simulink model "Aktuator"  (R2019b)
settings: Solver=FixedStepAuto  StartTime=0.0  StopTime=2  FixedStep=0.00001  RelTol=1e-3
values from neighbouring files (symbols this model uses):
  Drehzahlkonstante = 1070    [Init_Aktuator.m]    (also in Init_Aktuator_Klapp.m = 569; Init_Aktuator_Steuer.m)
  I_Konstante = 20    [Init_Aktuator.m]    (also in Init_Aktuator_Steuer.m)
  Moment_aero = 255.25    [Init_Aktuator.m]    (also in Init_Aktuator_Steuer.m)
  Momentenkonstante = 8.95/1000    (= 0.00895)    [Init_Aktuator.m]    (also in Init_Aktuator_Klapp.m = 0.0168; Init_Aktuator_Steuer.m)
  Motorreibkonstante = Reibmoment / (Leerlaufdrehzahl * 2 * pi / 60)    (= 3.47456064781e-06)    [Init_Aktuator.m]    (also in Init_Aktuator_Steuer.m)
  P_Konstante = 4    [Init_Aktuator.m]    (also in Init_Aktuator_Steuer.m)
  Reibung = 1    [Init_Aktuator.m]    (also in Init_Aktuator_Steuer.m)
  Sollwert0 = 20    [Init_Aktuator.m]    (also in Init_Aktuator_Steuer.m)
  Sollwert1 = -20    [Init_Aktuator.m]    (also in Init_Aktuator_Steuer.m)
  Sollwert2 = 0    [Init_Aktuator.m]    (also in Init_Aktuator_Steuer.m)
  Spannung = 12    [Init_Aktuator_Klapp.m]
  Spannung_max = Nennspannung * 2    (= 24)    [Init_Aktuator.m]    (also in Init_Aktuator_Steuer.m = 18)
  Startauslenkung = 0/180*pi    (= 0)    [Init_Aktuator.m]    (also in Init_Aktuator_Steuer.m)
  Steigung = 27.1*1000    (= 27100)    [Init_Aktuator.m]    (also in Init_Aktuator_Klapp.m = 0.002; Init_Aktuator_Steuer.m)
  t1 = Periodendauer/4    (= 0.1825)    [Init_Aktuator.m]    (also in Init_Aktuator_Steuer.m)
  t2 = Periodendauer * 3/4    (= 0.5475)    [Init_Aktuator.m]    (also in Init_Aktuator_Steuer.m)
  Traegheitsmoment_Getriebe = 0.005    [Init_Aktuator.m]    (also in Init_Aktuator_Steuer.m)
  Traegheitsmoment_GF = 0.054    [Init_Aktuator.m]    (also in Init_Aktuator_Steuer.m)
  Traegheitsmoment_Motor = 10.5/10000000    (= 1.05e-06)    [Init_Aktuator.m]    (also in Init_Aktuator_Steuer.m)
  Uebersetzung = 200    [Init_Aktuator.m]    (also in Init_Aktuator_Klapp.m = 3.7; Init_Aktuator_Steuer.m)
libraries: simulink x3
settings Model: Creator=Neu1  LastModifiedBy=Neu1

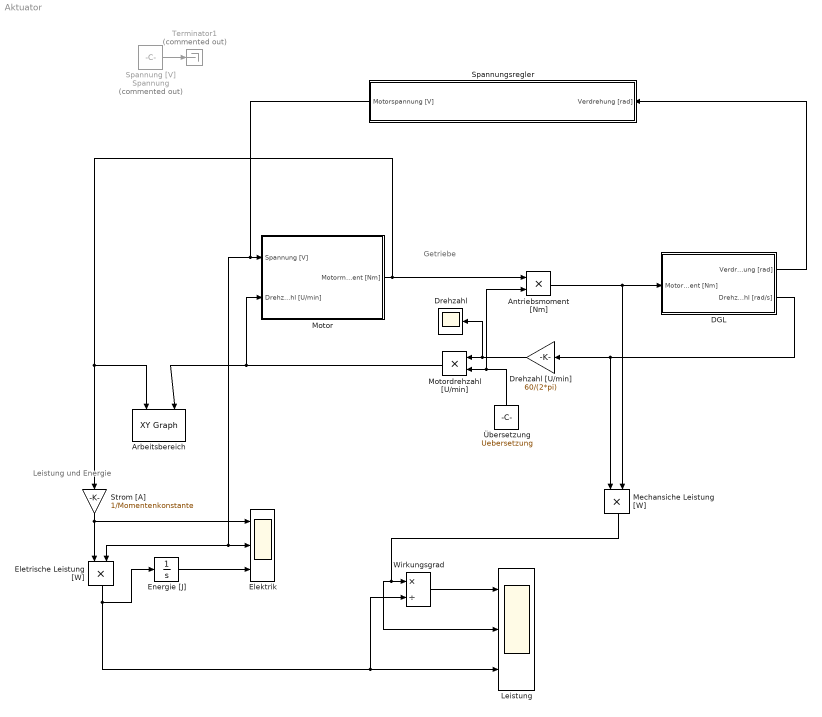
== system Aktuator ==
  note: Leistung und Energie
  note: Getriebe
  Antriebsmoment [Nm] : Product
  "Arbeitsbereich " : simulink/Sinks/XY Graph  xmin=-1  xmax=14  ymin=-1  ymax=3000  st=0.1
  DGL : Subsystem
  Drehzahl : Scope
  Drehzahl [U/min] : Gain  Gain=60/(2*pi)
  "Elektrik " : Scope  NumInputPorts=3
  Eletrische Leistung [W] : Product
  Energie [J] : Integrator
  Leistung : Scope  NumInputPorts=3
  "Mechansiche Leistung [W] " : Product
  Motor : Subsystem
  "Motordrehzahl [U/min] " : Product  Inputs=**
  Spannung [V] : Constant  Commented=on  Value=Spannung
  Spannungsregler : Subsystem
  Strom [A] : Gain  Gain=1/Momentenkonstante
  Terminator1 : Terminator  Commented=on
  Wirkungsgrad : Product  Inputs=*/
  Übersetzung : Constant  Value=Uebersetzung
  wires:
  Antriebsmoment [Nm]/1 -> "Mechansiche Leistung [W] "/2, DGL/1(Motormoment [Nm])
  Übersetzung/1 -> "Motordrehzahl [U/min] "/2, Antriebsmoment [Nm]/2
  "Mechansiche Leistung [W] "/1 -> Leistung/2, Wirkungsgrad/1
  Strom [A]/1 -> Eletrische Leistung [W]/1, "Elektrik "/1
  Eletrische Leistung [W]/1 -> Energie [J]/1, Leistung/3, Wirkungsgrad/2
  Wirkungsgrad/1 -> Leistung/1
  Energie [J]/1 -> "Elektrik "/3
  Spannung [V]/1 -> Terminator1/1
  "Motordrehzahl [U/min] "/1 -> Motor/2(Drehzahl [U/min]), "Arbeitsbereich "/2
  Motor/1(Motormoment [Nm]) -> "Arbeitsbereich "/1, Strom [A]/1, Antriebsmoment [Nm]/1
  Spannungsregler/1(Motorspannung [V]) -> "Elektrik "/2, Eletrische Leistung [W]/2, Motor/1(Spannung [V])
  DGL/1(Verdrehung [rad]) -> Spannungsregler/1(Verdrehung [rad])
  DGL/2(Drehzahl [rad/s]) -> "Mechansiche Leistung [W] "/1, Drehzahl [U/min]/1
  Drehzahl [U/min]/1 -> Drehzahl/1, "Motordrehzahl [U/min] "/1

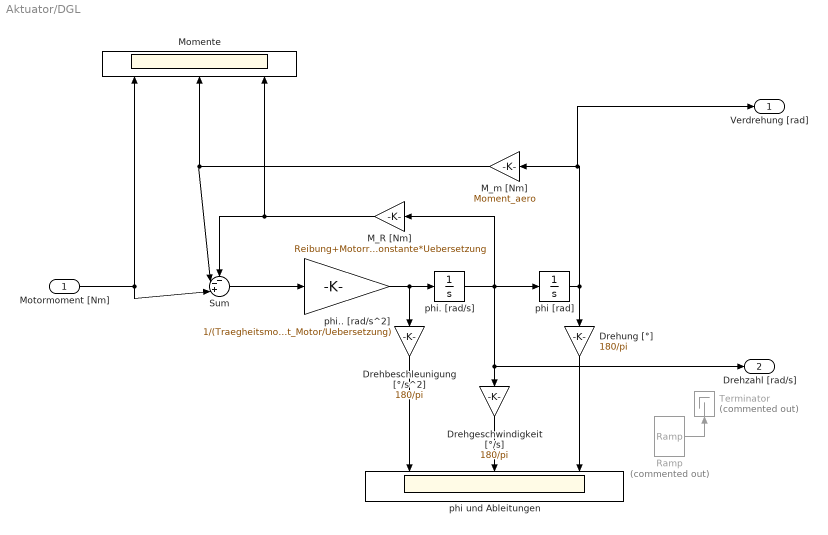
== system Aktuator/DGL ==
  Motormoment [Nm] : Inport
  Drehbeschleunigung [°/s^2] : Gain  Gain=180/pi
  Drehgeschwindigkeit [°/s] : Gain  Gain=180/pi
  Drehung [°] : Gain  Gain=180/pi
  M_R [Nm] : Gain  Gain=Reibung+Motorreibkonstante*Uebersetzung
  M_m [Nm] : Gain  Gain=Moment_aero
  Momente : Scope  NumInputPorts=3
  Ramp : simulink/Sources/Ramp  Commented=on  slope=6250  start=0  InitialOutput=0
  Sum : Sum  Inputs=--+|
  Terminator : Terminator  Commented=on
  phi [rad] : Integrator  InitialCondition=Startauslenkung  WrapState=on
  phi und Ableitungen : Scope  NumInputPorts=3
  phi. [rad/s] : Integrator
  phi.. [rad/s^2] : Gain  Gain=1/(Traegheitsmoment_GF+Traegheitsmoment_Getriebe+Traegheitsmoment_Motor/Uebersetzung)
  Verdrehung [rad] : Outport
  Drehzahl [rad/s] : Outport  Port=2
  wires:
  Sum/1 -> phi.. [rad/s^2]/1
  phi [rad]/1 -> Drehung [°]/1, Verdrehung [rad]/1, M_m [Nm]/1
  Ramp/1 -> Terminator/1
  Drehung [°]/1 -> phi und Ableitungen/3
  phi.. [rad/s^2]/1 -> phi. [rad/s]/1, Drehbeschleunigung [°/s^2]/1
  Drehgeschwindigkeit [°/s]/1 -> phi und Ableitungen/2
  M_m [Nm]/1 -> Sum/2, Momente/2
  Drehbeschleunigung [°/s^2]/1 -> phi und Ableitungen/1
  M_R [Nm]/1 -> Sum/1, Momente/3
  Motormoment [Nm]/1 -> Sum/3, Momente/1
  phi. [rad/s]/1 -> Drehzahl [rad/s]/1, Drehgeschwindigkeit [°/s]/1, M_R [Nm]/1, phi [rad]/1

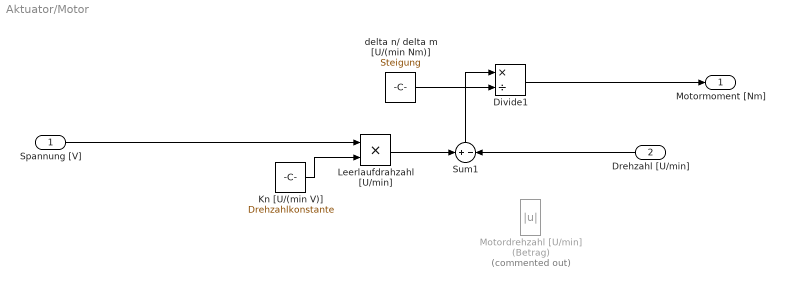
== system Aktuator/Motor ==
  Spannung [V] : Inport
  Drehzahl [U/min] : Inport  Port=2
  Divide1 : Product  Inputs=*/
  Kn [U/(min V)] : Constant  Value=Drehzahlkonstante
  Leerlaufdrahzahl [U/min] : Product
  Motordrehzahl [U/min] (Betrag) : Abs  Commented=on
  Sum1 : Sum  Inputs=+|-
  delta n/ delta m [U/(min Nm)] : Constant  Value=Steigung
  Motormoment [Nm] : Outport
  wires:
  delta n/ delta m [U/(min Nm)]/1 -> Divide1/2
  Sum1/1 -> Divide1/1
  Divide1/1 -> Motormoment [Nm]/1
  Spannung [V]/1 -> Leerlaufdrahzahl [U/min]/1
  Leerlaufdrahzahl [U/min]/1 -> Sum1/1
  Kn [U/(min V)]/1 -> Leerlaufdrahzahl [U/min]/2
  Drehzahl [U/min]/1 -> Sum1/2

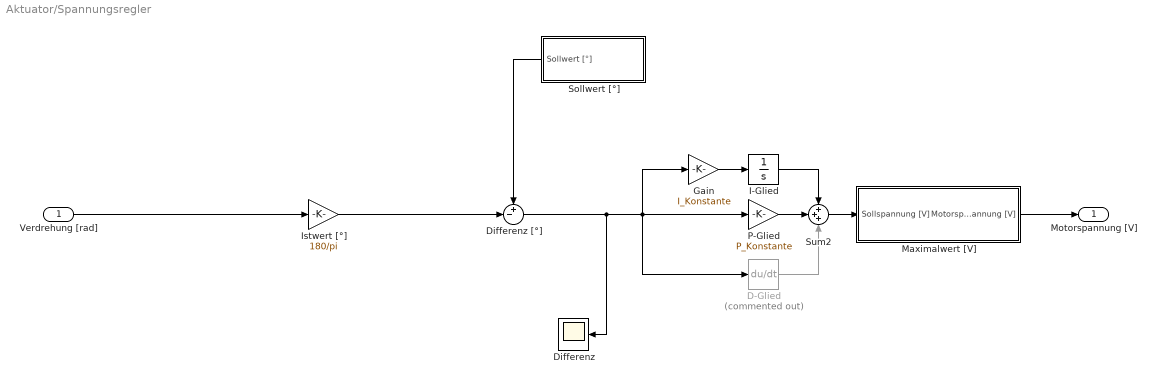
== system Aktuator/Spannungsregler ==
  Verdrehung [rad] : Inport
  D-Glied : Derivative  Commented=on  CoefficientInTFapproximation=D_Konstante
  Differenz : Scope
  Differenz [°] : Sum  Inputs=+-|
  Gain : Gain  Gain=I_Konstante
  I-Glied : Integrator
  Istwert [°] : Gain  Gain=180/pi
  Maximalwert [V] : Subsystem
  P-Glied : Gain  Gain=P_Konstante
  Sollwert [°] : Subsystem
  Sum2 : Sum  Inputs=+++
  Motorspannung [V] : Outport
  wires:
  Sum2/1 -> Maximalwert [V]/1("Sollspannung [V] ")
  Gain/1 -> I-Glied/1
  D-Glied/1 -> Sum2/3
  Differenz [°]/1 -> Gain/1, P-Glied/1, D-Glied/1, Differenz/1
  P-Glied/1 -> Sum2/2
  Sollwert [°]/1(Sollwert [°]) -> Differenz [°]/1
  I-Glied/1 -> Sum2/1
  Istwert [°]/1 -> Differenz [°]/2
  Verdrehung [rad]/1 -> Istwert [°]/1
  Maximalwert [V]/1("Motorspannung [V] ") -> Motorspannung [V]/1

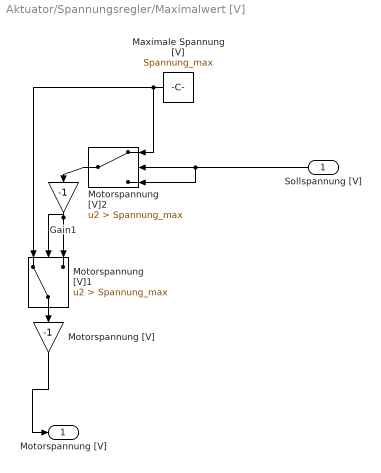
== system Aktuator/Spannungsregler/Maximalwert [V] ==
  "Sollspannung [V] " : Inport
  Gain1 : Gain  Gain=-1
  Maximale Spannung [V] : Constant  Value=Spannung_max
  Motorspannung [V] : Gain  Gain=-1
  Motorspannung [V]1 : Switch  Criteria=u2 > Threshold  Threshold=Spannung_max
  Motorspannung [V]2 : Switch  Criteria=u2 > Threshold  Threshold=Spannung_max
  "Motorspannung [V] " : Outport
  wires:
  Motorspannung [V]2/1 -> Gain1/1
  Gain1/1 -> Motorspannung [V]1/2, Motorspannung [V]1/3
  "Sollspannung [V] "/1 -> Motorspannung [V]2/3, Motorspannung [V]2/2
  Maximale Spannung [V]/1 -> Motorspannung [V]1/1, Motorspannung [V]2/1
  Motorspannung [V]1/1 -> Motorspannung [V]/1
  Motorspannung [V]/1 -> "Motorspannung [V] "/1

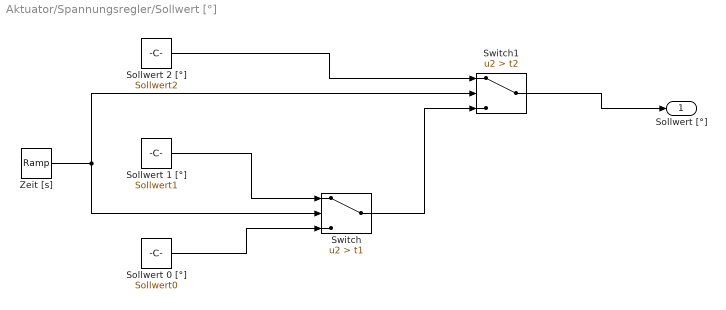
== system Aktuator/Spannungsregler/Sollwert [°] ==
  Sollwert 0 [°] : Constant  Value=Sollwert0
  Sollwert 1 [°] : Constant  Value=Sollwert1
  Sollwert 2 [°] : Constant  Value=Sollwert2
  Switch : Switch  Criteria=u2 > Threshold  Threshold=t1
  Switch1 : Switch  Criteria=u2 > Threshold  Threshold=t2
  Zeit [s] : simulink/Sources/Ramp  slope=1  start=0  InitialOutput=0
  Sollwert [°] : Outport
  wires:
  Switch1/1 -> Sollwert [°]/1
  Zeit [s]/1 -> Switch/2, Switch1/2
  Switch/1 -> Switch1/3
  Sollwert 1 [°]/1 -> Switch/1
  Sollwert 0 [°]/1 -> Switch/3
  Sollwert 2 [°]/1 -> Switch1/1
